simulink model "global_to_lokal"  (R2024b)
settings: Solver=VariableStepAuto  StartTime=0.0  StopTime=1000.0  RelTol=1e-3
settings Model: Creator=klyx  LastModifiedBy=klyx

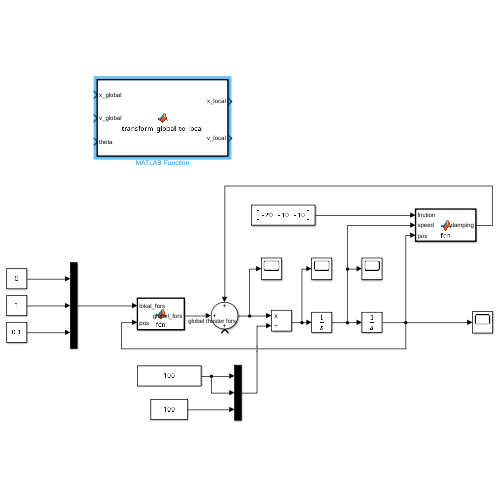
[thumbnail: Simulink's stored preview of the top-level diagram]
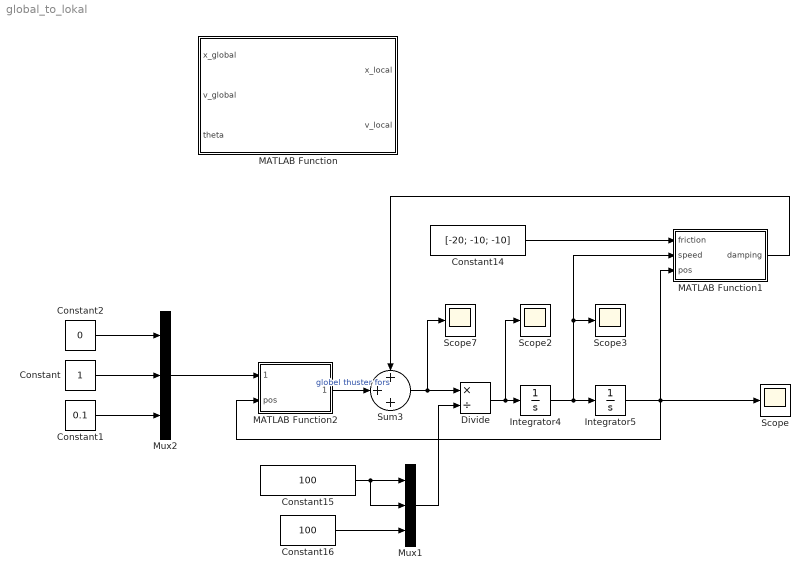
== system global_to_lokal ==
  Constant : Constant
  Constant1 : Constant  Value=0.1
  Constant14 : Constant  Value=[-20; -10; -10]
  Constant15 : Constant  Value=100
  Constant16 : Constant  Value=100
  Constant2 : Constant  Value=0
  Divide : Product  Inputs=*/
  Integrator4 : Integrator  InitialCondition=[10; 10; 0]
  Integrator5 : Integrator  InitialCondition=[0; 0; 1]
  MATLAB Function : MATLAB Function  TreatAsAtomicUnit=on
  MATLAB Function1 : MATLAB Function  TreatAsAtomicUnit=on
  MATLAB Function2 : MATLAB Function  TreatAsAtomicUnit=on
  Mux1 : Mux  Inputs=3
  Mux2 : Mux  Inputs=3
  Scope{,2..3,7} (4 alike) : Scope
  Sum3 : Sum  Inputs=+++
  wires:
  Constant/1 -> Mux2/2
  Constant2/1 -> Mux2/1
  Constant1/1 -> Mux2/3
  Mux2/1 -> MATLAB Function2/1(lokal_fors)
  Integrator5/1 -> MATLAB Function2/2(pos), Scope/1, MATLAB Function1/3(pos)
  Integrator4/1 -> Integrator5/1, Scope3/1, MATLAB Function1/2(speed)
  Divide/1 -> Scope2/1, Integrator4/1
  MATLAB Function1/1(damping) -> Sum3/1
  Sum3/1 -> Scope7/1, Divide/1
  Constant14/1 -> MATLAB Function1/1(friction)
  Constant15/1 -> Mux1/2, Mux1/1
  Constant16/1 -> Mux1/3
  Mux1/1 -> Divide/2
  MATLAB Function2/1(globel_fors) -> Sum3/2  "globel thuster fors"

== matlab function global_to_lokal/MATLAB Function1 ==
  data: friction input; damping output; speed input; pos input
function damping = fcn(friction, speed, pos)

firk = [friction(1) 0           0           ;
        0           friction(2) 0           ;
        0           0           friction(3)];

glo_to_lok = [cos(-pos(3)) -sin(-pos(3)) 0 ;
              sin(-pos(3)) cos(-pos(3))  0 ;
              0           0              1];

%s = speed
%rotl = inv(glo_to_lok)*firk*glo_to_lok;
damping = inv(glo_to_lok)*firk*glo_to_lok*speed;

== matlab function global_to_lokal/MATLAB Function ==
  data: x_global input; x_local output; v_global input; theta input; v_local output
function [x_local, v_local] = transform_global_to_local(x_global, v_global, theta)
    % Rotation matrix
    R = [cos(theta), -sin(theta), 0;
         sin(theta),  cos(theta), 0;
         0,          0,         1];

    % Transform global position & velocity to local frame
    x_local = R' * x_global; 
    v_local = R' * v_global;
end

== matlab function global_to_lokal/MATLAB Function2 ==
  data: lokal_fors input; globel_fors output; pos input
function globel_fors = fcn(lokal_fors ,pos)

xy_pos = [lokal_fors(1);lokal_fors(2)];

glo_to_lok = [cos(pos(3)) -sin(pos(3));
              sin(pos(3)) cos(pos(3))];

gb_xy_fors = inv(glo_to_lok)*xy_pos;

globel_fors  = [gb_xy_fors(1);gb_xy_fors(2); lokal_fors(3)];
